simulink model "electromagnet_a"  (R2024a)
settings: Solver=VariableStepAuto  StartTime=0.0  StopTime=te  MaxStep=te/100  RelTol=1e-3
values from neighbouring files (symbols this model uses):
  L = 44.15e-3    (= 0.04415)    [Electromagnet_par.m]    (also in coil_ironcore.m = 1; sim21_ODE.m = 1)
  R = 6.5    [Electromagnet_par.m]    (also in coil_ironcore.m = 10; sim21_ODE.m = 10)
  U = 10    [Electromagnet_par.m]    (also in coil_ironcore.m = 163; sim21_ODE.m = 230*sqrt(2))
  w = 2*pi/0.1    (= 62.8318530718)    [Electromagnet_par.m]    (also in coil_ironcore.m = 314.159265359; sim21_ODE.m = [0.5 1 2])
settings Model: Creator=ocean  LastModifiedBy=ocean

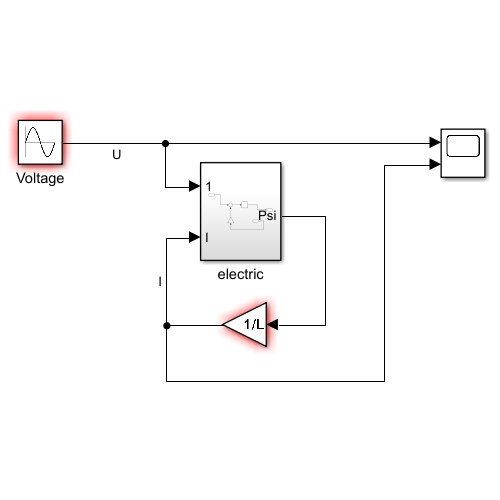
[thumbnail: Simulink's stored preview of the top-level diagram]
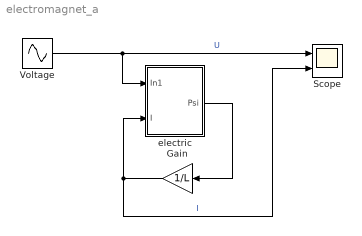
== system electromagnet_a ==
  Gain : Gain  Gain=1/L
  Scope : Scope  NumInputPorts=2
  Voltage : Sin  Amplitude=U  Frequency=w  SampleTime=0
  electric : Subsystem
  wires:
  Gain/1 -> Scope/2, electric/2(I)  "I"
  Voltage/1 -> electric/1(In1), Scope/1  "U"
  electric/1(Psi) -> Gain/1

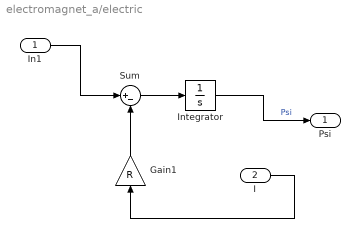
== system electromagnet_a/electric ==
  In1 : Inport
  I : Inport  Port=2
  Gain1 : Gain  Gain=R
  Integrator : Integrator
  Sum : Sum  Inputs=|+-
  Psi : Outport
  wires:
  Gain1/1 -> Sum/2
  Sum/1 -> Integrator/1
  I/1 -> Gain1/1
  In1/1 -> Sum/1
  Integrator/1 -> Psi/1  "Psi"
